simulink model "ploop_load"  (R2022b)
settings: Solver=ode15s  StartTime=0.0  StopTime=5  RelTol=1e-3  EnableMultiTasking=on
undefined symbols (not defined in the file): hp6, InertiaA, InertiaS, q_end, q_start, torq_const, torq_max
libraries: roblocks x12
settings Model: Creator=pic  LastModifiedBy=iarte
settings SolverCC: AlgebraicLoopSolver=TrustRegion
settings DataIOCC: SaveFormat=Array  SignalLoggingSaveFormat=ModelDataLogs  TimeSaveName=t  OutputSaveName=y  OutputOption=SpecifiedOutputTimes  OutputTimes=[0:0.001:1]'
settings OptimizationCC: ExpressionDepthLimit=2147483647  LifeSpan=inf
settings DebuggingCC: UnderspecifiedInitializationDetection=Classic  MergeDetectMultiDrivingBlocksExec=none  SolverPrmCheckMsg=warning  UnconnectedInputMsg=warning  UnconnectedOutputMsg=warning  UnconnectedLineMsg=warning  AllowSymbolicDim=off  StateNameClashWarn=warning  SFUnexpectedBacktrackingDiag=warning  SFNoUnconditionalDefaultTransitionDiag=warning  SFExecutionAtInitializationDiag=none  SFMachineParentedDataDiag=warning  ArithmeticOperatorsInVariantConditions=warning
settings HardwareCC: ProdBitPerPointer=32  ProdBitPerSizeT=32  ProdBitPerPtrDiffT=32  ProdLargestAtomicFloat=None  ProdIntDivRoundTo=Undefined  ProdEndianess=Unspecified  ProdWordSize=32  ProdHWDeviceType=32-bit Generic
settings ModelReferenceCC: EnableRefExpFcnMdlSchedulingChecks=on  PropagateSignalLabelsOutOfModel=off
settings SFSimCC: SimUseLocalCustomCode=off  CustomCodeUndefinedFunction=UseInterfaceOnly
settings RTWCC: RTWUseLocalCustomCode=off
settings CodeAppCC: StateflowObjectComments=on
settings GRTTargetCC: TargetLangStandard=C89/C90 (ANSI)  CombineOutputUpdateFcns=off  GRTInterface=on
settings ConfigComp: CovMetricSettings=dw  CovSaveCumulativeToWorkspaceVar=on  CovSaveSingleToWorkspaceVar=on  CovExternalEMLEnable=off  CovSFcnEnable=off

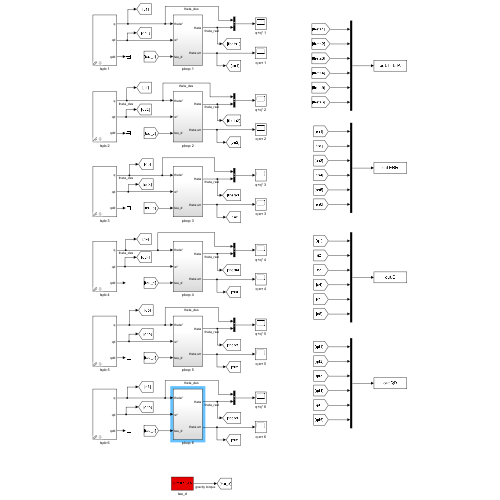
[thumbnail: Simulink's stored preview of the top-level diagram]
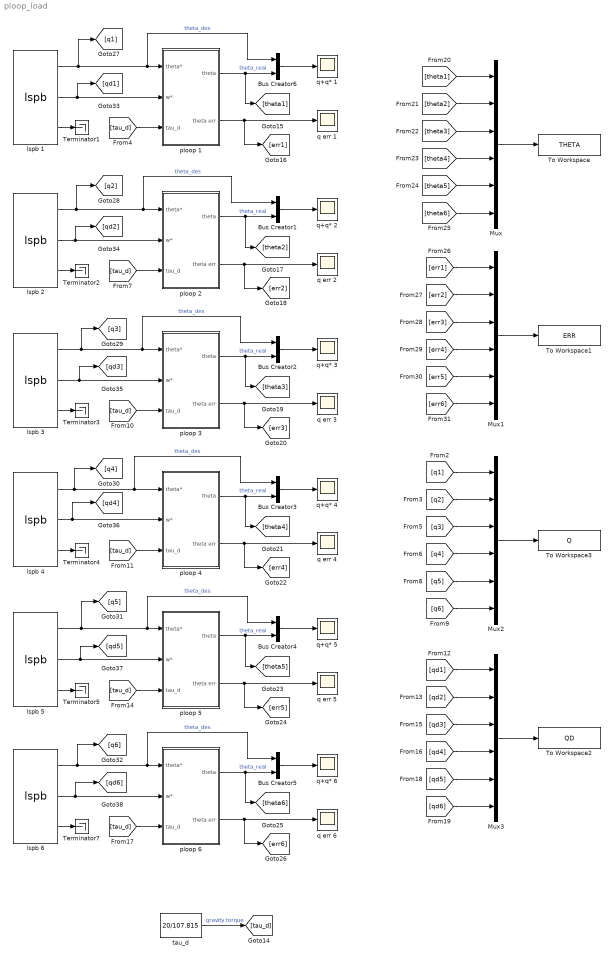
== system ploop_load ==
  Bus Creator{1..6} (6 alike) : BusCreator  Inputs=2
  Mux{,1..3} (4 alike) : Mux  Inputs=6
  Terminator{1..5,7} (6 alike) : Terminator
  To Workspace : ToWorkspace  VariableName=THETA  SaveFormat=Timeseries  SampleTime=-1
  To Workspace1 : ToWorkspace  VariableName=ERR  SaveFormat=Timeseries  SampleTime=-1
  To Workspace2 : ToWorkspace  VariableName=QD  SaveFormat=Timeseries  SampleTime=-1
  To Workspace3 : ToWorkspace  VariableName=Q  SaveFormat=Timeseries  SampleTime=-1
  lspb 1 : roblocks/Toolbox/lspb  q0=q_start(1)  qf=q_end(1)  tmax=stop_time
  lspb 2 : roblocks/Toolbox/lspb  q0=q_start(2)  qf=q_end(2)  tmax=stop_time
  lspb 3 : roblocks/Toolbox/lspb  q0=q_start(3)  qf=q_end(3)  tmax=stop_time
  lspb 4 : roblocks/Toolbox/lspb  q0=q_start(4)  qf=q_end(4)  tmax=stop_time
  lspb 5 : roblocks/Toolbox/lspb  q0=q_start(5)  qf=q_end(5)  tmax=stop_time
  lspb 6 : roblocks/Toolbox/lspb  q0=q_start(6)  qf=q_end(6)  tmax=stop_time
  ploop 1 : Subsystem
  ploop 2 : Subsystem
  ploop 3 : Subsystem
  ploop 4 : Subsystem
  ploop 5 : Subsystem
  ploop 6 : Subsystem
  q err {1..6} (6 alike) : Scope
  q+q* {1..6} (6 alike) : Scope
  tau_d : Constant  Value=20/107.815
  wires:
  Bus Creator2/1 -> q+q* 3/1
  ploop 4/2(theta err) -> q err 4/1, [err4]
  lspb 5/3 -> Terminator5/1
  lspb 6/3 -> Terminator7/1
  [q6] -> Mux2/6
  Mux/1 -> To Workspace/1
  lspb 3/1 -> [q3], Bus Creator2/1, ploop 3/1(theta*)  "theta_des"
  [theta5] -> Mux/5
  lspb 4/3 -> Terminator4/1
  [tau_d] -> ploop 6/3(tau_d)
  lspb 4/2 -> ploop 4/2(w*), [qd4]
  lspb 4/1 -> [q4], Bus Creator3/1, ploop 4/1(theta*)  "theta_des"
  ploop 2/2(theta err) -> q err 2/1, [err2]
  ploop 3/1(theta) -> [theta3], Bus Creator2/2  "theta_real"
  [err2] -> Mux1/2
  ploop 5/1(theta) -> [theta5], Bus Creator4/2  "theta_real"
  lspb 2/3 -> Terminator2/1
  [err5] -> Mux1/5
  tau_d/1 -> [tau_d]  "gravity torque"
  [theta6] -> Mux/6
  [err3] -> Mux1/3
  [tau_d] -> ploop 3/3(tau_d)
  lspb 5/1 -> [q5], Bus Creator4/1, ploop 5/1(theta*)  "theta_des"
  [err1] -> Mux1/1
  lspb 1/2 -> [qd1], ploop 1/2(w*)
  [q5] -> Mux2/5
  lspb 5/2 -> [qd5], ploop 5/2(w*)
  [theta4] -> Mux/4
  [theta3] -> Mux/3
  ploop 5/2(theta err) -> [err5], q err 5/1
  lspb 3/3 -> Terminator3/1
  ploop 2/1(theta) -> Bus Creator1/2, [theta2]  "theta_real"
  lspb 6/2 -> [qd6], ploop 6/2(w*)
  Bus Creator5/1 -> q+q* 6/1
  Bus Creator3/1 -> q+q* 4/1
  lspb 2/2 -> [qd2], ploop 2/2(w*)
  [theta1] -> Mux/1
  ploop 1/2(theta err) -> [err1], q err 1/1
  Mux1/1 -> To Workspace1/1
  ploop 3/2(theta err) -> [err3], q err 3/1
  Bus Creator6/1 -> q+q* 1/1
  lspb 1/1 -> [q1], Bus Creator6/1, ploop 1/1(theta*)  "theta_des"
  [tau_d] -> ploop 4/3(tau_d)
  ploop 6/2(theta err) -> q err 6/1, [err6]
  [qd2] -> Mux3/2
  [tau_d] -> ploop 5/3(tau_d)
  [q3] -> Mux2/3
  ploop 6/1(theta) -> Bus Creator5/2, [theta6]  "theta_real"
  [theta2] -> Mux/2
  [q4] -> Mux2/4
  Bus Creator4/1 -> q+q* 5/1
  [qd6] -> Mux3/6
  lspb 1/3 -> Terminator1/1
  [qd5] -> Mux3/5
  [qd3] -> Mux3/3
  ploop 4/1(theta) -> Bus Creator3/2, [theta4]  "theta_real"
  [qd4] -> Mux3/4
  lspb 2/1 -> [q2], Bus Creator1/1, ploop 2/1(theta*)  "theta_des"
  Bus Creator1/1 -> q+q* 2/1
  [qd1] -> Mux3/1
  ploop 1/1(theta) -> [theta1], Bus Creator6/2  "theta_real"
  lspb 6/1 -> [q6], ploop 6/1(theta*), Bus Creator5/1  "theta_des"
  [tau_d] -> ploop 2/3(tau_d)
  [err6] -> Mux1/6
  Mux2/1 -> To Workspace3/1
  Mux3/1 -> To Workspace2/1
  lspb 3/2 -> [qd3], ploop 3/2(w*)
  [q2] -> Mux2/2
  [err4] -> Mux1/4
  [tau_d] -> ploop 1/3(tau_d)
  [q1] -> Mux2/1

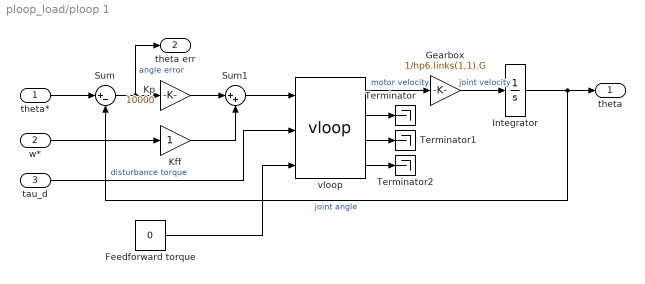
== system ploop_load/ploop 1 ==
  theta* : Inport
  w* : Inport  Port=2
  tau_d : Inport  Port=3
  Feedforward torque : Constant  Value=0
  Gearbox : Gain  Gain=1/hp6.links(1,1).G
  Integrator : Integrator  InitialCondition=q_start(1)
  Kff : Gain
  Kp : Gain  Gain=10000
  Sum : Sum  Inputs=|+-
  Sum1 : Sum  Inputs=|++
  Terminator : Terminator
  Terminator1 : Terminator
  Terminator2 : Terminator
  vloop : roblocks/Arm/vloop  J=InertiaA(1)  B=hp6.links(1,1).B  Km=torq_const(1)  tau_max=torq_max(1)  Kv=2  Ki=50  T=0.001
  theta : Outport  VectorParamsAs1DForOutWhenUnconnected=off
  theta err : Outport  Port=2  VectorParamsAs1DForOutWhenUnconnected=off
  wires:
  Gearbox/1 -> Integrator/1  "joint velocity"
  Feedforward torque/1 -> vloop/3
  tau_d/1 -> vloop/2  "disturbance torque"
  vloop/1 -> Gearbox/1  "motor velocity"
  vloop/4 -> Terminator2/1
  vloop/3 -> Terminator1/1
  vloop/2 -> Terminator/1
  Kff/1 -> Sum1/2
  w*/1 -> Kff/1
  Sum1/1 -> vloop/1
  Kp/1 -> Sum1/1
  theta*/1 -> Sum/1
  Integrator/1 -> Sum/2, theta/1  "joint angle"
  Sum/1 -> theta err/1, Kp/1  "angle error"

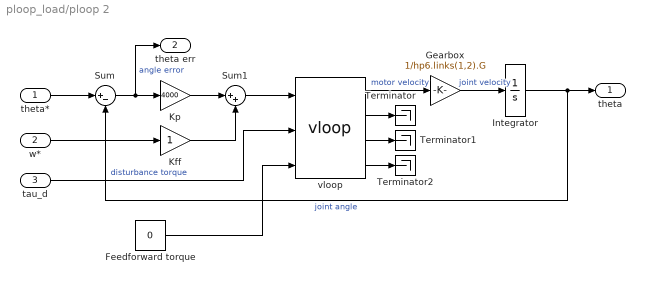
== system ploop_load/ploop 2 ==
  theta* : Inport
  w* : Inport  Port=2
  tau_d : Inport  Port=3
  Feedforward torque : Constant  Value=0
  Gearbox : Gain  Gain=1/hp6.links(1,2).G
  Integrator : Integrator  InitialCondition=q_start(2)
  Kff : Gain
  Kp : Gain  Gain=4000
  Sum : Sum  Inputs=|+-
  Sum1 : Sum  Inputs=|++
  Terminator : Terminator
  Terminator1 : Terminator
  Terminator2 : Terminator
  vloop : roblocks/Arm/vloop  J=InertiaS(2)  B=hp6.links(1,2).B  Km=torq_const(2)  tau_max=torq_max(2)  Kv=1.5  Ki=50  T=0.001
  theta : Outport  VectorParamsAs1DForOutWhenUnconnected=off
  theta err : Outport  Port=2  VectorParamsAs1DForOutWhenUnconnected=off
  wires:
  Sum/1 -> Kp/1, theta err/1  "angle error"
  Integrator/1 -> theta/1, Sum/2  "joint angle"
  theta*/1 -> Sum/1
  Kp/1 -> Sum1/1
  Sum1/1 -> vloop/1
  w*/1 -> Kff/1
  Kff/1 -> Sum1/2
  vloop/2 -> Terminator/1
  vloop/3 -> Terminator1/1
  vloop/4 -> Terminator2/1
  vloop/1 -> Gearbox/1  "motor velocity"
  tau_d/1 -> vloop/2  "disturbance torque"
  Feedforward torque/1 -> vloop/3
  Gearbox/1 -> Integrator/1  "joint velocity"

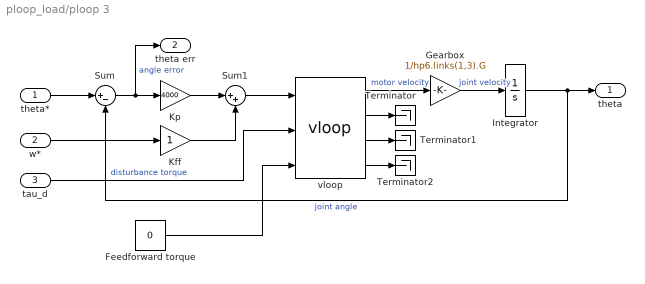
== system ploop_load/ploop 3 ==
  theta* : Inport
  w* : Inport  Port=2
  tau_d : Inport  Port=3
  Feedforward torque : Constant  Value=0
  Gearbox : Gain  Gain=1/hp6.links(1,3).G
  Integrator : Integrator  InitialCondition=q_start(3)
  Kff : Gain
  Kp : Gain  Gain=4000
  Sum : Sum  Inputs=|+-
  Sum1 : Sum  Inputs=|++
  Terminator : Terminator
  Terminator1 : Terminator
  Terminator2 : Terminator
  vloop : roblocks/Arm/vloop  J=InertiaS(3)  B=hp6.links(1,3).B  Km=torq_const(3)  tau_max=torq_max(3)  Kv=2  Ki=80  T=0.001
  theta : Outport  VectorParamsAs1DForOutWhenUnconnected=off
  theta err : Outport  Port=2  VectorParamsAs1DForOutWhenUnconnected=off
  wires:
  Gearbox/1 -> Integrator/1  "joint velocity"
  Feedforward torque/1 -> vloop/3
  tau_d/1 -> vloop/2  "disturbance torque"
  vloop/1 -> Gearbox/1  "motor velocity"
  vloop/4 -> Terminator2/1
  vloop/3 -> Terminator1/1
  vloop/2 -> Terminator/1
  Kff/1 -> Sum1/2
  w*/1 -> Kff/1
  Sum1/1 -> vloop/1
  Kp/1 -> Sum1/1
  theta*/1 -> Sum/1
  Integrator/1 -> Sum/2, theta/1  "joint angle"
  Sum/1 -> theta err/1, Kp/1  "angle error"

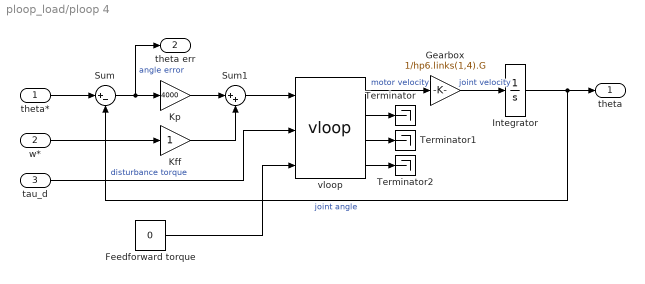
== system ploop_load/ploop 4 ==
  theta* : Inport
  w* : Inport  Port=2
  tau_d : Inport  Port=3
  Feedforward torque : Constant  Value=0
  Gearbox : Gain  Gain=1/hp6.links(1,4).G
  Integrator : Integrator  InitialCondition=q_start(4)
  Kff : Gain
  Kp : Gain  Gain=4000
  Sum : Sum  Inputs=|+-
  Sum1 : Sum  Inputs=|++
  Terminator : Terminator
  Terminator1 : Terminator
  Terminator2 : Terminator
  vloop : roblocks/Arm/vloop  J=InertiaS(4)  B=hp6.links(1,4).B  Km=torq_const(4)  tau_max=torq_max(4)  Kv=0.09  Ki=9  T=0.001
  theta : Outport  VectorParamsAs1DForOutWhenUnconnected=off
  theta err : Outport  Port=2  VectorParamsAs1DForOutWhenUnconnected=off
  wires:
  Sum/1 -> Kp/1, theta err/1  "angle error"
  Integrator/1 -> theta/1, Sum/2  "joint angle"
  theta*/1 -> Sum/1
  Kp/1 -> Sum1/1
  Sum1/1 -> vloop/1
  w*/1 -> Kff/1
  Kff/1 -> Sum1/2
  vloop/2 -> Terminator/1
  vloop/3 -> Terminator1/1
  vloop/4 -> Terminator2/1
  vloop/1 -> Gearbox/1  "motor velocity"
  tau_d/1 -> vloop/2  "disturbance torque"
  Feedforward torque/1 -> vloop/3
  Gearbox/1 -> Integrator/1  "joint velocity"

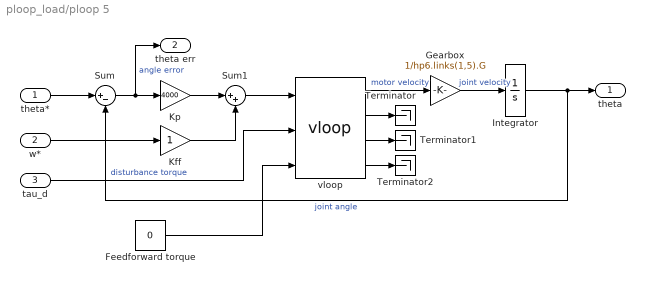
== system ploop_load/ploop 5 ==
  theta* : Inport
  w* : Inport  Port=2
  tau_d : Inport  Port=3
  Feedforward torque : Constant  Value=0
  Gearbox : Gain  Gain=1/hp6.links(1,5).G
  Integrator : Integrator  InitialCondition=q_start(5)
  Kff : Gain
  Kp : Gain  Gain=4000
  Sum : Sum  Inputs=|+-
  Sum1 : Sum  Inputs=|++
  Terminator : Terminator
  Terminator1 : Terminator
  Terminator2 : Terminator
  vloop : roblocks/Arm/vloop  J=InertiaS(5)  B=hp6.links(1,5).B  Km=torq_const(5)  tau_max=torq_max(5)  Kv=0.1  Ki=10  T=0.001
  theta : Outport  VectorParamsAs1DForOutWhenUnconnected=off
  theta err : Outport  Port=2  VectorParamsAs1DForOutWhenUnconnected=off
  wires:
  Gearbox/1 -> Integrator/1  "joint velocity"
  Feedforward torque/1 -> vloop/3
  tau_d/1 -> vloop/2  "disturbance torque"
  vloop/1 -> Gearbox/1  "motor velocity"
  vloop/4 -> Terminator2/1
  vloop/3 -> Terminator1/1
  vloop/2 -> Terminator/1
  Kff/1 -> Sum1/2
  w*/1 -> Kff/1
  Sum1/1 -> vloop/1
  Kp/1 -> Sum1/1
  theta*/1 -> Sum/1
  Integrator/1 -> Sum/2, theta/1  "joint angle"
  Sum/1 -> theta err/1, Kp/1  "angle error"

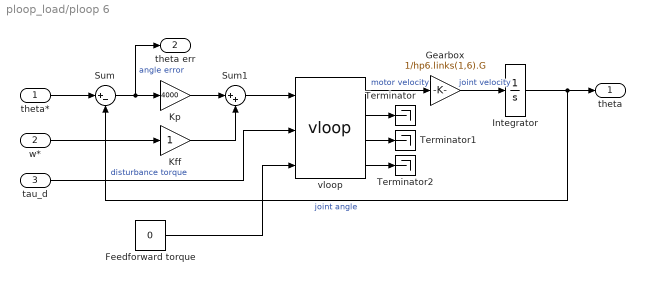
== system ploop_load/ploop 6 ==
  theta* : Inport
  w* : Inport  Port=2
  tau_d : Inport  Port=3
  Feedforward torque : Constant  Value=0
  Gearbox : Gain  Gain=1/hp6.links(1,6).G
  Integrator : Integrator  InitialCondition=q_start(6)
  Kff : Gain
  Kp : Gain  Gain=4000
  Sum : Sum  Inputs=|+-
  Sum1 : Sum  Inputs=|++
  Terminator : Terminator
  Terminator1 : Terminator
  Terminator2 : Terminator
  vloop : roblocks/Arm/vloop  J=InertiaS(6)  B=hp6.links(1,6).B  Km=torq_const(6)  tau_max=torq_max(6)  Kv=0.1  Ki=10  T=0.001
  theta : Outport  VectorParamsAs1DForOutWhenUnconnected=off
  theta err : Outport  Port=2  VectorParamsAs1DForOutWhenUnconnected=off
  wires:
  Sum/1 -> Kp/1, theta err/1  "angle error"
  Integrator/1 -> theta/1, Sum/2  "joint angle"
  theta*/1 -> Sum/1
  Kp/1 -> Sum1/1
  Sum1/1 -> vloop/1
  w*/1 -> Kff/1
  Kff/1 -> Sum1/2
  vloop/2 -> Terminator/1
  vloop/3 -> Terminator1/1
  vloop/4 -> Terminator2/1
  vloop/1 -> Gearbox/1  "motor velocity"
  tau_d/1 -> vloop/2  "disturbance torque"
  Feedforward torque/1 -> vloop/3
  Gearbox/1 -> Integrator/1  "joint velocity"
